simulink model "Q_2_2_SS_Control_with_Robust_Tracking"  (R2024b)
settings: Solver=ode45  StartTime=0.0  StopTime=20  FixedStep=0.001  RelTol=1e-3
InitFcn:
  | load_params_inertial_case
  | SS_Calculations
  | RUN
values from neighbouring files (symbols this model uses):
  delta_c = 1 / sqrt(2)    [PID_calculations.m]    (also in SS_Calculations.m)
  Ke = place(Ae, Be, poles)    [SS_Calculations.m]
  Nx_aug = [0; Nx]    [SS_Calculations.m]
  w_c = 2 * pi * 20    (= 125.663706144)    [PID_calculations.m]    (also in SS_Calculations.m)
undefined symbols (not defined in the file or in its folder): gbox, KIe, Nre, Nue, rads2rpm, sens
settings Model: Creator=JS  LastModifiedBy=JS

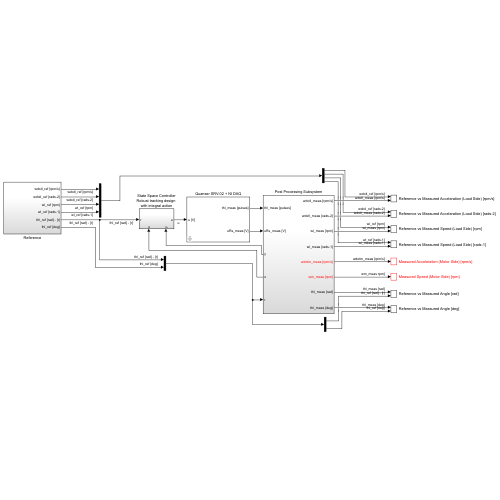
[thumbnail: Simulink's stored preview of the top-level diagram]
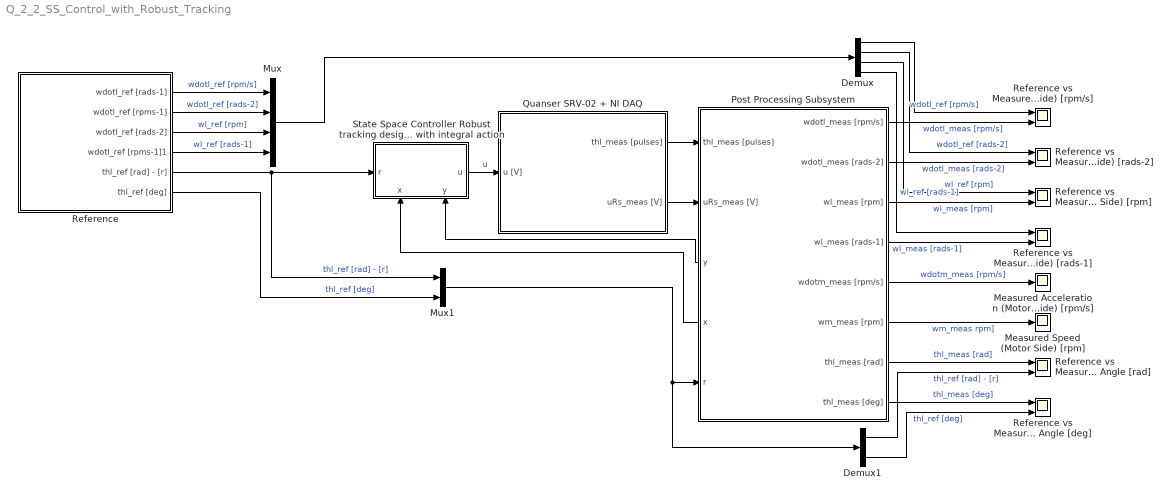
== system Q_2_2_SS_Control_with_Robust_Tracking ==
  Demux : Demux
  Demux1 : Demux  Outputs=2
  Measured Acceleration (Motor Side) [rpm/s] : Scope
  Measured Speed (Motor Side) [rpm] : Scope
  Mux : Mux
  Mux1 : Mux  Inputs=2
  Post Processing Subsystem : Subsystem
      settings: PortSchema="{\"entries\":[{\"content\":{\"sides\":[{\"content\":{\"connectorIds\":[\"In1\",\"In2\",\"Out9\",\"Out10\",\"In3\"]},\"type\":\"ConnectorPlacement.EquallySpacedRectSide\",\"uuid\":\"fbb4e644-04bd-4e71-aa0b-cfc387bbb09a\"},{\"content\":{\"connectorIds\":[\"Out1\",\"Out2\",\"Out3\",\"Out4\",\"Out5\",\"Out6\",\"Out7\",\"Out8\"],\"side\":\"RIGHT\"},\"type\":\"ConnectorPlacement.EquallySpacedRectSide\",\"uuid\":\"dd064039-a21a-4a3c-8ef8-fe4f48a2450d\"},{\"content\":{\"side\":\"TOP\"},\"type\":\"ConnectorPlacement.EquallySpacedRectSide\",\"uuid\":\"822d5d45-3d41-4c7c-b419-3ed51d05db8c\"},{\"content\":{\"side\":\"BOTTOM\"},\"type\":\"ConnectorPlacement.EquallySpacedRectSide\",\"uuid\":\"54449d93-ef3e-40ea-aebb-85c8031ea2fb\"}]},\"type\":\"ConnectorPlacement.EquallySpacedConnector\",\"uuid\":\"92e7ab69-1beb-4a77-8126-06820b7739a0\"}],\"packageUris\":[\"http://schema.mathworks.com/mf0/Connector/R2020b\"],\"version\":\"1.0\"}"
  Quanser SRV-02 + NI DAQ : Subsystem  mask(Quanser SRV-02 (with inertial load) + NI DAQ){Ts=0.001, fricType=Coulomb + viscous}
      mask prompts: Ts "NI DAQ Sample Time:"; fricType "Friction model"
      mask help: Quanser SRV-02 (with inertial load) + NI DAQ model.
      mask init:
      | %%  Sensors data
      | 
      | %   shunt resistor
      | sens.curr.Rs = 0.5;                         %   resistance [Ohm]   
      | sens.curr.uRs_std = 0.01;                   %   voltage noise standard dev [V]                           
      | sens.curr.uRs_var = sens.curr.uRs_std^2;	%   voltage noise variance [V^2]
      | 
      | %   Hewlett-Packard HEDS-5540#A06 optical encoder
      | sens.enc.ppr = 500*4;                       %   pulses per rotation
      | sens.enc.pulse2deg = 360/sens.enc.ppr;      %   [pulses] -> [deg]
      | sens.enc.pulse2rad = 2*pi/sens.enc.ppr;     %   [pulses] -> [rad]
      | sens.enc.deg2pulse = sens.enc.ppr/360;      %   [deg] -> [pulses]
      | sens.enc.rad2pulse = sens.enc.ppr/2/pi;     %   [rad] -> [pulses]
      | 
      | 
      | %%  Data acquisition board (daq) data
      | 
      | %   NI PCI-6221 DAC data
      | daq.dac.bits = 16;                                  %   resolution (bits)
      | daq.dac.fs   = 10;                                  %   full scale 
      | daq.dac.q    = 2*daq.dac.fs/(2^daq.dac.bits-1);     %	quantization
      | 
      | %   NI PCI-6221 ADC data
      | daq.adc.bits = 16;                                  %   resolution (bits)
      | daq.adc.fs   = 10;                                  %   full scale (as set in SLDRT Analog Input block)
      | daq.adc.q    = 2*daq.adc.fs/(2^daq.adc.bits-1);     %   quantization
      mask Help:
      | Riccardo Antonello (antonello@dei.unipd.it)
      | 
      | April 24, 2020
      | 
      | Dept. of Information Engineering, University of Padova
      mask TypeOptions fricType: Coulomb + viscous | Karnopp
  Reference : Subsystem
  Reference vs Measured Acceleration (Load Side) [rads-2] : Scope  NumInputPorts=2
  Reference vs Measured Acceleration (Load Side) [rpm/s] : Scope  NumInputPorts=2
  "Reference vs Measured Angle [deg] " : Scope  NumInputPorts=2
  "Reference vs Measured Angle [rad] " : Scope  NumInputPorts=2
  Reference vs Measured Speed (Load Side) [rads-1] : Scope  NumInputPorts=2
  Reference vs Measured Speed (Load Side) [rpm] : Scope  NumInputPorts=2
  State Space Controller Robust tracking design with integral action : Subsystem
      settings: PortSchema="{\"entries\":[{\"content\":{\"sides\":[{\"content\":{\"connectorIds\":[\"In1\"]},\"type\":\"ConnectorPlacement.EquallySpacedRectSide\",\"uuid\":\"74d9c870-2294-4822-a6d3-4399bc83e7e5\"},{\"content\":{\"connectorIds\":[\"Out1\"],\"side\":\"RIGHT\"},\"type\":\"ConnectorPlacement.EquallySpacedRectSide\",\"uuid\":\"6f81acdf-9ee7-44fd-b558-ba6528172edd\"},{\"content\":{\"side\":\"TOP\"},\"type\":\"ConnectorPlacement.EquallySpacedRectSide\",\"uuid\":\"4f3d1ea1-d8bf-4f70-af12-87bbcb1fce4f\"},{\"content\":{\"connectorIds\":[\"In2\",\"In3\"],\"side\":\"BOTTOM\"},\"type\":\"ConnectorPlacement.EquallySpacedRectSide\",\"uuid\":\"9156a720-a385-4025-8862-c6f7bccb4ba0\"}]},\"type\":\"ConnectorPlacement.EquallySpacedConnector\",\"uuid\":\"cab39010-31fb-45c0-a7ca-94e81f26881b\"}],\"packageUris\":[\"http://schema.mathworks.com/mf0/Connector/R2020b\"],\"version\":\"1.0\"}"
  wires:
  Reference/5(thl_ref [rad] - [r]) -> Mux1/1, State Space Controller Robust tracking design with integral action/1(r)  "thl_ref [rad] - [r]"
  Reference/2(wdotl_ref [rpms-1]) -> Mux/2  "wdotl_ref [rads-2]"
  Reference/1(wdotl_ref [rads-1]) -> Mux/1  "wdotl_ref [rpm/s]"
  Reference/6(thl_ref [deg]) -> Mux1/2  "thl_ref [deg]"
  State Space Controller Robust tracking design with integral action/1(u) -> Quanser SRV-02 + NI DAQ/1(u [V])  "u"
  Quanser SRV-02 + NI DAQ/1(thl_meas [pulses]) -> Post Processing Subsystem/1(thl_meas [pulses])
  Quanser SRV-02 + NI DAQ/2(uRs_meas [V]) -> Post Processing Subsystem/2(uRs_meas [V])
  Post Processing Subsystem/1(wdotl_meas [rpm/s]) -> Reference vs Measured Acceleration (Load Side) [rpm/s]/2  "wdotl_meas [rpm/s]"
  Post Processing Subsystem/8(thl_meas [deg]) -> "Reference vs Measured Angle [deg] "/1  "thl_meas [deg]"
  Post Processing Subsystem/7(thl_meas [rad]) -> "Reference vs Measured Angle [rad] "/1  "thl_meas [rad]"
  Post Processing Subsystem/2(wdotl_meas [rads-2]) -> Reference vs Measured Acceleration (Load Side) [rads-2]/2  "wdotl_meas [rads-2]"
  Post Processing Subsystem/10(x) -> State Space Controller Robust tracking design with integral action/2(x)
  Post Processing Subsystem/5(wdotm_meas [rpm/s]) -> Measured Acceleration (Motor Side) [rpm/s]/1  "wdotm_meas [rpm/s]"
  Post Processing Subsystem/6(wm_meas [rpm]) -> Measured Speed (Motor Side) [rpm]/1  "wm_meas rpm]"
  Post Processing Subsystem/4(wl_meas [rads-1]) -> Reference vs Measured Speed (Load Side) [rads-1]/2  "wl_meas [rads-1]"
  Post Processing Subsystem/3(wl_meas [rpm]) -> Reference vs Measured Speed (Load Side) [rpm]/2  "wl_meas [rpm]"
  Reference/3(wdotl_ref [rads-2]) -> Mux/3  "wl_ref [rpm]"
  Reference/4(wdotl_ref [rpms-1]1) -> Mux/4  "wl_ref [rads-1]"
  Demux/1 -> Reference vs Measured Acceleration (Load Side) [rpm/s]/1  "wdotl_ref [rpm/s]"
  Demux/2 -> Reference vs Measured Acceleration (Load Side) [rads-2]/1  "wdotl_ref [rads-2]"
  Demux/3 -> Reference vs Measured Speed (Load Side) [rpm]/1  "wl_ref [rpm]"
  Demux/4 -> Reference vs Measured Speed (Load Side) [rads-1]/1  "wl_ref [rads-1]"
  Mux/1 -> Demux/1
  Mux1/1 -> Post Processing Subsystem/3(r), Demux1/1
  Demux1/1 -> "Reference vs Measured Angle [rad] "/2  "thl_ref [rad] - [r]"
  Demux1/2 -> "Reference vs Measured Angle [deg] "/2  "thl_ref [deg]"
  Post Processing Subsystem/9(y) -> State Space Controller Robust tracking design with integral action/3(y)

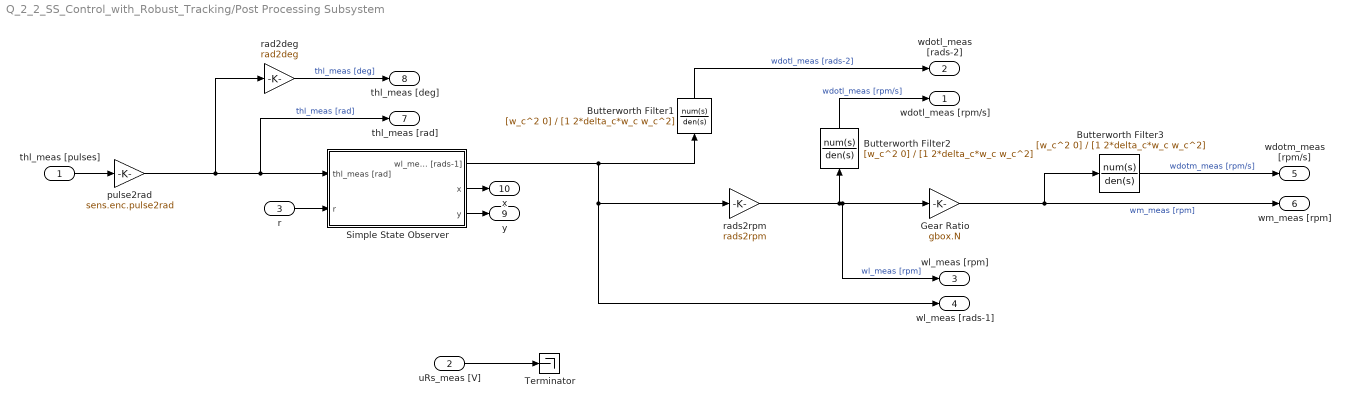
== system Q_2_2_SS_Control_with_Robust_Tracking/Post Processing Subsystem ==
  thl_meas [pulses] : Inport
  uRs_meas [V] : Inport  Port=2
  r : Inport  Port=3
  Butterworth Filter1 : TransferFcn  Numerator=[w_c^2 0]  Denominator=[1 2*delta_c*w_c w_c^2]
  Butterworth Filter2 : TransferFcn  Numerator=[w_c^2 0]  Denominator=[1 2*delta_c*w_c w_c^2]
  Butterworth Filter3 : TransferFcn  Numerator=[w_c^2 0]  Denominator=[1 2*delta_c*w_c w_c^2]
  Gear Ratio : Gain  Gain=gbox.N
  Simple State Observer : Subsystem
  Terminator : Terminator
  pulse2rad : Gain  Gain=sens.enc.pulse2rad
  rad2deg : Gain  Gain=rad2deg
  rads2rpm : Gain  Gain=rads2rpm
  wdotl_meas [rpm/s] : Outport
  wdotl_meas [rads-2] : Outport  Port=2
  wl_meas [rpm] : Outport  Port=3
  wl_meas [rads-1] : Outport  Port=4
  wdotm_meas [rpm/s] : Outport  Port=5
  wm_meas [rpm] : Outport  Port=6
  thl_meas [rad] : Outport  Port=7
  thl_meas [deg] : Outport  Port=8
  y : Outport  Port=9
  x : Outport  Port=10
  wires:
  pulse2rad/1 -> rad2deg/1, thl_meas [rad]/1, Simple State Observer/1(thl_meas [rad])  "thl_meas [rad]"
  rad2deg/1 -> thl_meas [deg]/1  "thl_meas [deg]"
  uRs_meas [V]/1 -> Terminator/1
  thl_meas [pulses]/1 -> pulse2rad/1
  Butterworth Filter3/1 -> wdotm_meas [rpm/s]/1  "wdotm_meas [rpm/s]"
  Butterworth Filter2/1 -> wdotl_meas [rpm/s]/1  "wdotl_meas [rpm/s]"
  rads2rpm/1 -> Gear Ratio/1, wl_meas [rpm]/1, Butterworth Filter2/1  "wl_meas [rpm]"
  Butterworth Filter1/1 -> wdotl_meas [rads-2]/1  "wdotl_meas [rads-2]"
  Gear Ratio/1 -> wm_meas [rpm]/1, Butterworth Filter3/1  "wm_meas [rpm]"
  Simple State Observer/1(wl_meas [rads-1]) -> rads2rpm/1, wl_meas [rads-1]/1, Butterworth Filter1/1
  Simple State Observer/2(x) -> x/1
  Simple State Observer/3(y) -> y/1
  r/1 -> Simple State Observer/2(r)

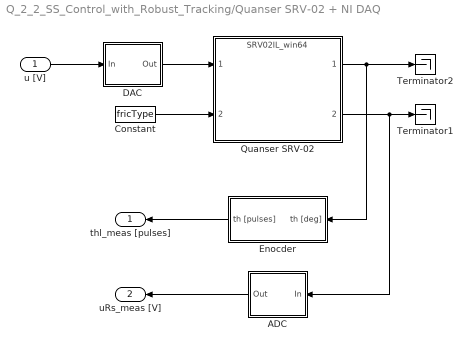
== system Q_2_2_SS_Control_with_Robust_Tracking/Quanser SRV-02 + NI DAQ ==
  u [V] : Inport
  ADC : Subsystem
  Constant : Constant  Value=fricType
  DAC : Subsystem
  Enocder : Subsystem
  Quanser SRV-02 : ModelReference  ModelNameDialog=SRV02IL_win64.slxp  ModelReferenceVersion=1.44  CopyOfModelProtected=on
  Terminator1 : Terminator
  Terminator2 : Terminator
  thl_meas [pulses] : Outport
  uRs_meas [V] : Outport  Port=2
  wires:
  Enocder/1(th [pulses]) -> thl_meas [pulses]/1
  ADC/1(Out) -> uRs_meas [V]/1
  DAC/1(Out) -> Quanser SRV-02/1
  Quanser SRV-02/2 -> ADC/1(In), Terminator1/1
  u [V]/1 -> DAC/1(In)
  Quanser SRV-02/1 -> Enocder/1(th [deg]), Terminator2/1
  Constant/1 -> Quanser SRV-02/2

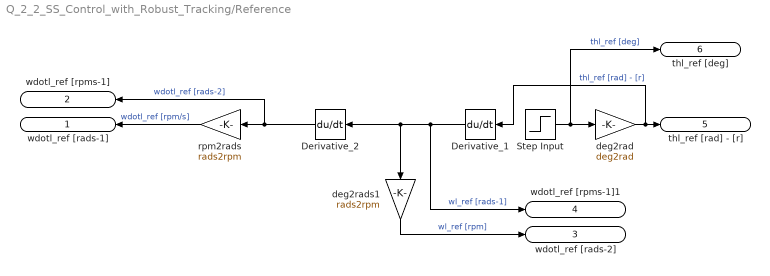
== system Q_2_2_SS_Control_with_Robust_Tracking/Reference ==
  Derivative_1 : Derivative
  Derivative_2 : Derivative
  Step Input : Step  Time=0  After=70  SampleTime=0
  deg2rad : Gain  Gain=deg2rad
  deg2rads1 : Gain  Gain=rads2rpm
  rpm2rads : Gain  Gain=rads2rpm
  wdotl_ref [rads-1] : Outport
  wdotl_ref [rpms-1] : Outport  Port=2
  wdotl_ref [rads-2] : Outport  Port=3
  wdotl_ref [rpms-1]1 : Outport  Port=4
  thl_ref [rad] - [r] : Outport  Port=5
  thl_ref [deg] : Outport  Port=6
  wires:
  deg2rad/1 -> Derivative_1/1, thl_ref [rad] - [r]/1  "thl_ref [rad] - [r]"
  Step Input/1 -> thl_ref [deg]/1, deg2rad/1  "thl_ref [deg]"
  Derivative_2/1 -> rpm2rads/1, wdotl_ref [rpms-1]/1  "wdotl_ref [rads-2]"
  rpm2rads/1 -> wdotl_ref [rads-1]/1  "wdotl_ref [rpm/s]"
  Derivative_1/1 -> Derivative_2/1, deg2rads1/1, wdotl_ref [rpms-1]1/1  "wl_ref [rads-1]"
  deg2rads1/1 -> wdotl_ref [rads-2]/1  "wl_ref [rpm]"

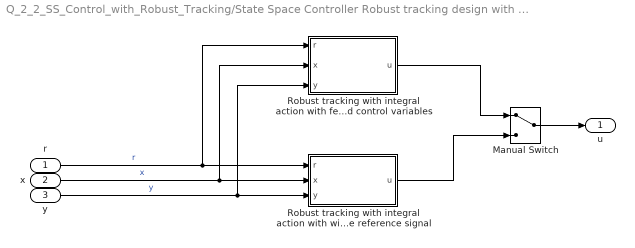
== system Q_2_2_SS_Control_with_Robust_Tracking/State Space Controller Robust tracking design with integral action ==
  r : Inport
  x : Inport  Port=2
  y : Inport  Port=3
  "  Robust tracking with integral action with feedforward action on state and control variables" : Subsystem
  " Robust tracking with integral action with with feedforward compensation of the reference signal" : Subsystem
  Manual Switch : ManualSwitch
  u : Outport
  wires:
  x/1 -> "  Robust tracking with integral action with feedforward action on state and control variables"/2(x), " Robust tracking with integral action with with feedforward compensation of the reference signal"/2(x)  "x"
  r/1 -> "  Robust tracking with integral action with feedforward action on state and control variables"/1(r), " Robust tracking with integral action with with feedforward compensation of the reference signal"/1(r)  "r"
  "  Robust tracking with integral action with feedforward action on state and control variables"/1(u) -> Manual Switch/1
  " Robust tracking with integral action with with feedforward compensation of the reference signal"/1(u) -> Manual Switch/2
  Manual Switch/1 -> u/1
  y/1 -> "  Robust tracking with integral action with feedforward action on state and control variables"/3(y), " Robust tracking with integral action with with feedforward compensation of the reference signal"/3(y)  "y"

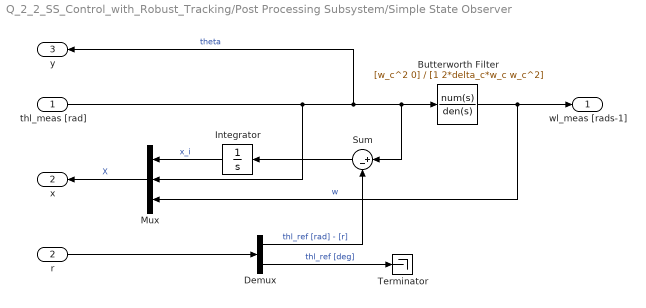
== system Q_2_2_SS_Control_with_Robust_Tracking/Post Processing Subsystem/Simple State Observer ==
  thl_meas [rad] : Inport
  r : Inport  Port=2
  Butterworth Filter : TransferFcn  Numerator=[w_c^2 0]  Denominator=[1 2*delta_c*w_c w_c^2]
  Demux : Demux  Outputs=2
  Integrator : Integrator
  Mux : Mux  Inputs=3
  Sum : Sum  Inputs=|+-
  Terminator : Terminator
  wl_meas [rads-1] : Outport
  x : Outport  Port=2
  y : Outport  Port=3
  wires:
  thl_meas [rad]/1 -> Mux/2, Sum/1, Butterworth Filter/1, y/1  "theta"
  Butterworth Filter/1 -> Mux/3, wl_meas [rads-1]/1  "w"
  Mux/1 -> x/1  "X"
  Demux/2 -> Terminator/1  "thl_ref [deg]"
  Demux/1 -> Sum/2  "thl_ref [rad] - [r]"
  r/1 -> Demux/1
  Sum/1 -> Integrator/1
  Integrator/1 -> Mux/1  "x_i"

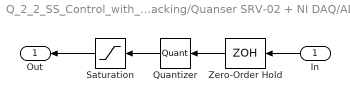
== system Q_2_2_SS_Control_with_Robust_Tracking/Quanser SRV-02 + NI DAQ/ADC ==
  In : Inport
  Quantizer : Quantizer  QuantizationInterval=daq.adc.q
  Saturation : Saturate  UpperLimit=daq.adc.fs  LowerLimit=-daq.adc.fs
  Zero-Order Hold : ZeroOrderHold  SampleTime=Ts
  Out : Outport
  wires:
  Saturation/1 -> Out/1
  In/1 -> Zero-Order Hold/1
  Quantizer/1 -> Saturation/1
  Zero-Order Hold/1 -> Quantizer/1

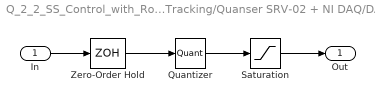
== system Q_2_2_SS_Control_with_Robust_Tracking/Quanser SRV-02 + NI DAQ/DAC ==
  In : Inport
  Quantizer : Quantizer  QuantizationInterval=daq.dac.q
  Saturation : Saturate  UpperLimit=daq.dac.fs  LowerLimit=-daq.dac.fs
  Zero-Order Hold : ZeroOrderHold  SampleTime=Ts
  Out : Outport
  wires:
  Quantizer/1 -> Saturation/1
  In/1 -> Zero-Order Hold/1
  Zero-Order Hold/1 -> Quantizer/1
  Saturation/1 -> Out/1

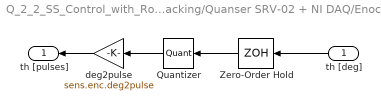
== system Q_2_2_SS_Control_with_Robust_Tracking/Quanser SRV-02 + NI DAQ/Enocder ==
  th [deg] : Inport
  Quantizer : Quantizer  QuantizationInterval=sens.enc.pulse2deg
  Zero-Order Hold : ZeroOrderHold  SampleTime=Ts
  deg2pulse : Gain  Gain=sens.enc.deg2pulse
  th [pulses] : Outport
  wires:
  Quantizer/1 -> deg2pulse/1
  th [deg]/1 -> Zero-Order Hold/1
  Zero-Order Hold/1 -> Quantizer/1
  deg2pulse/1 -> th [pulses]/1

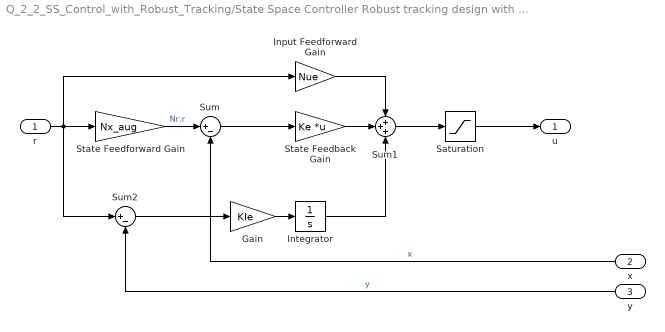
== system Q_2_2_SS_Control_with_Robust_Tracking/State Space Controller Robust tracking design with integral action/  Robust tracking with integral action with feedforward action on state and control variables ==
  r : Inport
  x : Inport  Port=2
  y : Inport  Port=3
  Gain : Gain  Gain=KIe
  Input Feedforward Gain : Gain  Gain=Nue
  Integrator : Integrator
  Saturation : Saturate  UpperLimit=10  LowerLimit=-10
  State Feedback Gain : Gain  Gain=Ke  Multiplication=Matrix(K*u)
  State Feedforward Gain : Gain  Gain=Nx_aug
  Sum : Sum  Inputs=|+-
  Sum1 : Sum  Inputs=+++
  Sum2 : Sum  Inputs=|+-
  u : Outport
  wires:
  r/1 -> Sum2/1, Input Feedforward Gain/1, State Feedforward Gain/1
  State Feedforward Gain/1 -> Sum/1  "Nr.r"
  Sum1/1 -> Saturation/1
  State Feedback Gain/1 -> Sum1/2
  Input Feedforward Gain/1 -> Sum1/1
  x/1 -> Sum/2  "x"
  Saturation/1 -> u/1
  Gain/1 -> Integrator/1
  y/1 -> Sum2/2  "y"
  Sum2/1 -> Gain/1
  Integrator/1 -> Sum1/3
  Sum/1 -> State Feedback Gain/1

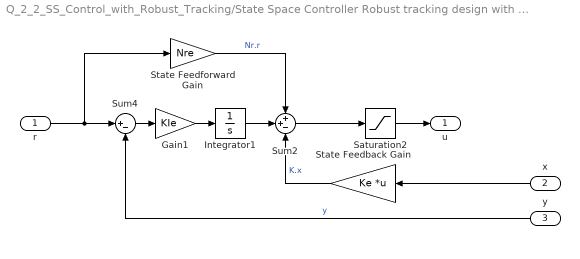
== system Q_2_2_SS_Control_with_Robust_Tracking/State Space Controller Robust tracking design with integral action/ Robust tracking with integral action with with feedforward compensation of the reference signal ==
  r : Inport
  x : Inport  Port=2
  y : Inport  Port=3
  Gain1 : Gain  Gain=KIe
  Integrator1 : Integrator
  Saturation2 : Saturate  UpperLimit=10  LowerLimit=-10
  State Feedback Gain : Gain  Gain=Ke  Multiplication=Matrix(K*u)
  State Feedforward Gain : Gain  Gain=Nre
  Sum2 : Sum  Inputs=++-
  Sum4 : Sum  Inputs=|+-
  u : Outport
  wires:
  State Feedback Gain/1 -> Sum2/3  "K.x"
  Sum2/1 -> Saturation2/1
  Saturation2/1 -> u/1
  State Feedforward Gain/1 -> Sum2/1  "Nr.r"
  x/1 -> State Feedback Gain/1
  r/1 -> Sum4/1, State Feedforward Gain/1
  Gain1/1 -> Integrator1/1
  Integrator1/1 -> Sum2/2
  Sum4/1 -> Gain1/1
  y/1 -> Sum4/2  "y"
